simulink model "rlOvertakeTwoCars"  (R2022b)
settings: Solver=ode45  StartTime=0.0  StopTime=inf  FixedStep=0.001  RelTol=5e-3
PreLoadFcn:
  | setUpModel
PostLoadFcn:
  | setUpMain
model workspace (MAT data in the model file):
  firstWarning = 0
  originalScenarioChecksum = 'F73A6DA3C723D3CA73A6F931B7A52A9C'
values from neighbouring files (symbols this model uses):
  accel_vec = (-4:0.5:4)'    [setUpModel.m]
  amax = 3    [setUpMain.m]
  amin = -3    [setUpMain.m]
  dyNorm = [dyNorm 1.1]    [setUpSlipstream.m]
  e1_initial = 0    [setUpMain.m]
  e2_initial = 0    [setUpMain.m]
  L = data.ActorSpecifications.Length    [setUpModel.m]
  psi_o1 = 0.0058 * (pi/180)    (= 0.000101229096616)    [setUpModel.m]
  psi_o2 = 0.3528 *(pi/180)    (= 0.00615752160104)    [setUpModel.m]
  ry = [ry 0]    [setUpSlipstream.m]
  ssSwitch = 1    [setUpSlipstream.m]
  tolpsi = 10 * pi/180    (= 0.174532925199)    [setUpSlipstream.m]
  toly = 1.2*W /2    [setUpSlipstream.m]
  Ts = 0.1    [setUpMPC.m]
  TsRL = Ts    [setUpRLEnv.m]
  umax = 0.3    [setUpMain.m]
  umin = -0.3    [setUpMain.m]
  v_o1 = highSpeed1    (= 35)    [setUpModel.m]
  v_o2 = highSpeed2    (= 36)    [setUpModel.m]
  vel1 = highSpeed1 * ones(length(xlt),length(ylt))    [setUpModel.m]
  vel2 = highSpeed2 * ones(length(xlt),length(ylt))    [setUpModel.m]
  vel_vec = 0:2:20    [setUpModel.m]
  W = data.ActorSpecifications(1,1).Width    [setUpSlipstream.m]
  X_o1 = xRef1(1)    [setUpModel.m]
  X_o2 = xRef2(1)    [setUpModel.m]
  xFollow = [0 x1 xFollow 60]    [setUpSlipstream.m]
  xLead = [0 -x0 xLead]    [setUpSlipstream.m]
  xlt = -250:10:200    [setUpModel.m]
  Y_o1 = yRef1(1)    [setUpModel.m]
  Y_o2 = yRef2(1)    [setUpModel.m]
  yFollow = [c y1 yFollow 1]    [setUpSlipstream.m]
  yLead = [c y0 yLead]    [setUpSlipstream.m]
  ylt = -150:10:100    [setUpModel.m]
undefined symbols (not defined in the file or in its folder): curvature1, curvature2, deg, DiscIntNeverNeededParam, gradbp1, gradbp2, psi, rad, s, v_o, x_colpen, x_o, y_colpen, Z_colpen
libraries: simulink x26, autolibsharedcommon x22, autolibutils x10, autolibshared x10, vehdynlibtirecommon x8, drivingscenarioandsensors x4, autolibpowerinfoutils x4, sharedtransform x4, aerolibconvert2 x2, simulink_extras x2, vehdynlibtire x2, mpcadaslib x1
(part 1 of 8)
settings Model: PacingRate=0.700000  Creator=valakshe  LastModifiedBy=16koc1
settings SolverCC: AlgebraicLoopSolver=TrustRegion
settings DebuggingCC: UnconnectedInputMsg=warning  UnconnectedOutputMsg=warning  UnconnectedLineMsg=warning  SFMachineParentedDataDiag=warning
settings ModelReferenceCC: EnableRefExpFcnMdlSchedulingChecks=on
settings RTWCC: DLArmComputeVersion=19.05

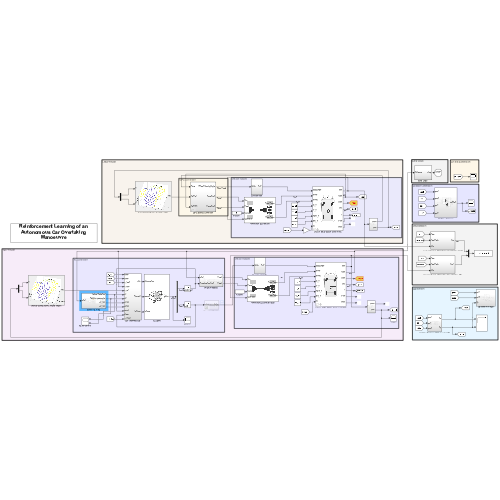
[thumbnail: Simulink's stored preview of the top-level diagram]
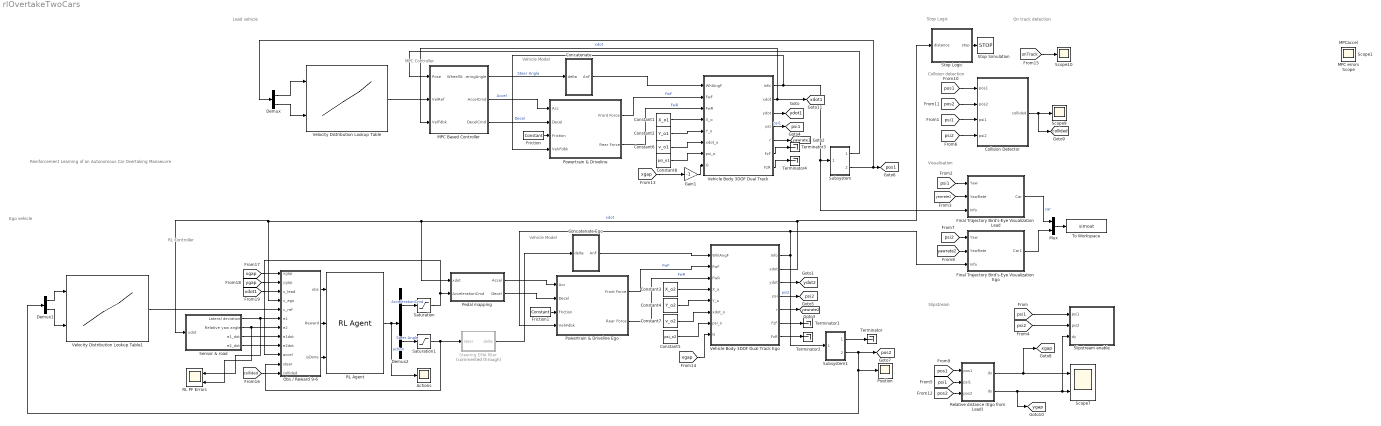
== system rlOvertakeTwoCars ==
  note: On track detection
  note: RL Controller
  note: Collision detection
  note: Slipstream
  note: Visualisation
  note: Ego vehicle
  note: Lead vehicle
  note: Stop Logic
  note: Vehicle Model
  note: Reinforcement Learning of an Autonomous Car Overtaking Manoeuvre
  note: MPC Controller
  note: Vehicle Model
  Actions : Scope
  Collision Detector : Subsystem
  Concatenate : Subsystem
  Concatenate Ego : Subsystem
  Constant1 : Constant  Value=X_o1
  Constant2 : Constant  Value=Y_o1
  Constant3 : Constant  Value=X_o2
  Constant4 : Constant  Value=Y_o2
  Constant5 : Constant  Value=psi_o2
  Constant6 : Constant  Value=v_o1
  Constant7 : Constant  Value=v_o2
  Constant8 : Constant  Value=psi_o1
  Demux : Demux  Outputs=2
  Demux1 : Demux  Outputs=2
  Demux2 : Demux  Outputs=2
  Final Trajectory Bird's-Eye Visualization Ego : Subsystem
  Final Trajectory Bird's-Eye Visualization Lead : Subsystem
  Friction : vehdynlibtirecommon/Constant  const=1.5  numWheels=4
  Friction1 : vehdynlibtirecommon/Constant  const=1.5  numWheels=4
  Gain1 : Gain  Gain=-1
  MPC Based Controller : Subsystem  AncestorBlock=rewardLibrary/MPC Based Controller  VariantControl=Stanley
      settings: LibrarySourceBlock=rewardLibrary/MPC Based Controller
  Mux : Mux  Inputs=2
  Obs / Reward 9-6 : Subsystem  AncestorBlock=rewardLibrary/Obs // Reward 6-2
      settings: LibrarySourceBlock=rewardLibrary/Obs // Reward 6-2
  Pedal mapping : Subsystem
  Position : Scope
  Powertrain & Driveline : Subsystem
      mask Display: image('vdbslibpt.png');
  Powertrain & Driveline Ego : Subsystem
      mask Display: image('vdbslibpt.png');
  RL Agent : rllib/RL Agent  Agent=agent  ExternalActionAsInput=off  ProvideLastAction=off  ProvideCumRwd=off  TreatAsDirectFeedthrough=on  UseStrictObservationDataTypes=off
  RL PF Errors : Scope  NumInputPorts=2
  Relative distance (Ego from Lead) : Subsystem
  Saturation : Saturate  UpperLimit=amax  LowerLimit=amin
  Saturation1 : Saturate  UpperLimit=umax  LowerLimit=umin
  Scope{,1,9..10} (4 alike) : Scope
  Scope7 : Scope  NumInputPorts=2
  Sensor & road : Subsystem
  Slipstream enable : Subsystem
  Steering EMA filter : Subsystem  Commented=through
  Stop Logic : Subsystem
  Stop Simulation : Stop
  Subsystem : Subsystem
  Subsystem1 : Subsystem
  Terminator{,1..4} (5 alike) : Terminator
  To Workspace : ToWorkspace  VariableName=simout  SaveFormat=Timeseries  SampleTime=-1
  Vehicle Body 3DOF Dual Track : Subsystem  AncestorBlock=autolibshared/Vehicle Body 3DOF Single Track  mask(Vehicle Body 3DOF Lateral){trackMode=Dual, inputMode=External forces, frontSteerMode=on, rearSteerMode=off, windMode=off, muMode=off, extFMode=off, extMMode=off, htchFMode=off, htchMMode=off, extXo=on, extpsio=on, extxdoto=on, extro=off, extYo=on, extTamb=off, extydoto=off, aMode=2, NF=2, NR=2, m=2000, a=1.4*4.7/3, b=1.6*4.7/3, h=0.35, dh=1, hh=0.2, X_o=0, xdot_o=v_o, CalphaMode=off, sigmaMode=on, d=0, hl=0, w=[1.4,1.4], Cy_f=12e3, Cy_r=11e3, sigma_f=.1, sigma_r=.1, alpha_f_brk=[-.1 .1], Cy_f_data=[-9e3 9e3], alpha_r_brk=[-.1 .1], Cy_r_data=[-9e3 9e3], Y_o=0, ydot_o=0, Izz=4000, psi_o=0, r_o=0, Af=2, Cd=.3, Cl=.1, Cpm=.1, beta_w=[0:0.01:0.3], Cs=[0:0.03:0.9], Cym=[0:0.01:0.3], Pabs=101325, Tair=273, g=9.81, mu=1, xdot_tol=.01, Fznom=5000, Fxtire_sat=7e4, Fytire_sat=7e4, longOff=0, latOff=0, vertOff=0, wrapAng=off}
      mask prompts: trackMode "autoblks_shared:autoblkVehBody3DofLat:blkPrm_trackMode"; inputMode "autoblks_shared:autoblkVehBody3DofLat:blkPrm_inputMode"; frontSteerMode "autoblks_shared:autoblkVehBody3DofLat:blkPrm_frontSteerMode"; rearSteerMode "autoblks_shared:autoblkVehBody3DofLat:blkPrm_rearSteerMode"; windMode "autoblks_shared:autoblkVehBody3DofLat:blkPrm_windMode"; muMode "autoblks_shared:autoblkVehBody3DofLat:blkPrm_muMode"; extFMode "autoblks_shared:autoblkVehBody3DofLat:blkPrm_extFMode"; extMMode "autoblks_shared:autoblkVehBody3DofLat:blkPrm_extMMode"; htchFMode "autoblks_shared:autoblkVehBody3DofLat:blkPrm_htchFMode"; htchMMode "autoblks_shared:autoblkVehBody3DofLat:blkPrm_htchMMode"; extXo "autoblks_shared:autoblkVehBody3DofLat:blkPrm_extXo"; extpsio "autoblks_shared:autoblkVehBody3DofLat:blkPrm_extpsio"; extxdoto "autoblks_shared:autoblkVehBody3DofLat:blkPrm_extxdoto"; extro "autoblks_shared:autoblkVehBody3DofLat:blkPrm_extro"; extYo "autoblks_shared:autoblkVehBody3DofLat:blkPrm_extYo"; extTamb "autoblks_shared:autoblkVehBody3DofLat:blkPrm_extTamb"; extydoto "autoblks_shared:autoblkVehBody3DofLat:blkPrm_extydoto"; NF "autoblks_shared:autoblkVehBody3DofLat:blkPrm_NF"; NR "autoblks_shared:autoblkVehBody3DofLat:blkPrm_NR"; m "autoblks_shared:autoblkVehBody3DofLat:blkPrm_m"; a "autoblks_shared:autoblkVehBody3DofLat:blkPrm_a"; b "autoblks_shared:autoblkVehBody3DofLat:blkPrm_b"; h "autoblks_shared:autoblkVehBody3DofLat:blkPrm_h"; dh "autoblks_shared:autoblkVehBody3DofLat:blkPrm_dh"; hh "autoblks_shared:autoblkVehBody3DofLat:blkPrm_hh"; X_o "autoblks_shared:autoblkVehBody3DofLat:blkPrm_X_o"; xdot_o "autoblks_shared:autoblkVehBody3DofLat:blkPrm_xdot_o"; CalphaMode "autoblks_shared:autoblkVehBody3DofLat:blkPrm_CalphaMode"; sigmaMode "autoblks_shared:autoblkVehBody3DofLat:blkPrm_sigmaMode"; d "autoblks_shared:autoblkVehBody3DofLat:blkPrm_d"; hl "autoblks_shared:autoblkVehBody3DofLat:blkPrm_hl"; w "autoblks_shared:autoblkVehBody3DofLat:blkPrm_w"; Cy_f "autoblks_shared:autoblkVehBody3DofLat:blkPrm_Cy_f"; Cy_r "autoblks_shared:autoblkVehBody3DofLat:blkPrm_Cy_r"; sigma_f "autoblks_shared:autoblkVehBody3DofLat:blkPrm_sigma_f"; sigma_r "autoblks_shared:autoblkVehBody3DofLat:blkPrm_sigma_r"; alpha_f_brk "autoblks_shared:autoblkVehBody3DofLat:blkPrm_alpha_f_brk"; Cy_f_data "autoblks_shared:autoblkVehBody3DofLat:blkPrm_Cy_f_data"; alpha_r_brk "autoblks_shared:autoblkVehBody3DofLat:blkPrm_alpha_r_brk"; Cy_r_data "autoblks_shared:autoblkVehBody3DofLat:blkPrm_Cy_r_data"; Y_o "autoblks_shared:autoblkVehBody3DofLat:blkPrm_Y_o"; ydot_o "autoblks_shared:autoblkVehBody3DofLat:blkPrm_ydot_o"; Izz "autoblks_shared:autoblkVehBody3DofLat:blkPrm_Izz"; psi_o "autoblks_shared:autoblkVehBody3DofLat:blkPrm_psi_o"; r_o "autoblks_shared:autoblkVehBody3DofLat:blkPrm_r_o"; Af "autoblks_shared:autoblkVehBody3DofLat:blkPrm_Af"; Cd "autoblks_shared:autoblkVehBody3DofLat:blkPrm_Cd"; Cl "autoblks_shared:autoblkVehBody3DofLat:blkPrm_Cl"; Cpm "autoblks_shared:autoblkVehBody3DofLat:blkPrm_Cpm"; beta_w "autoblks_shared:autoblkVehBody3DofLat:blkPrm_beta_w"; Cs "autoblks_shared:autoblkVehBody3DofLat:blkPrm_Cs"; Cym "autoblks_shared:autoblkVehBody3DofLat:blkPrm_Cym"; Pabs "autoblks_shared:autoblkVehBody3DofLat:blkPrm_Pabs"; Tair "autoblks_shared:autoblkVehBody3DofLat:blkPrm_Tair"; g "autoblks_shared:autoblkVehBody3DofLat:blkPrm_g"; mu "autoblks_shared:autoblkVehBody3DofLat:blkPrm_mu"; xdot_tol "autoblks_shared:autoblkVehBody3DofLat:blkPrm_xdot_tol"; Fznom "autoblks_shared:autoblkVehBody3DofLat:blkPrm_Fznom"; Fxtire_sat "autoblks_shared:autoblkVehBody3DofLat:blkPrm_Fxtire_sat"; Fytire_sat "autoblks_shared:autoblkVehBody3DofLat:blkPrm_Fytire_sat"; longOff "autoblks_shared:autoblkVehBody3DofLat:blkPrm_longOff"; latOff "autoblks_shared:autoblkVehBody3DofLat:blkPrm_latOff"; vertOff "autoblks_shared:autoblkVehBody3DofLat:blkPrm_vertOff"; wrapAng "autoblks_shared:autoblkVehBody3DofLat:blkPrm_wrapAng"
      mask help: autoblks_shared:autoblkVehBody3DofLat:blkDesc
      mask init:
      | [~]=autosharedicon('vehdynliblat3dof',gcb,0);
      settings: LibrarySourceBlock=autolibshared/Vehicle Body 3DOF Single Track
      mask Help: eval('autosharedhelp(''vb3doflat'')');
      mask TypeOptions trackMode: autoblks_shared:autoblkVehBody3DofLat:blkCmb_trackMode_c1 | autoblks_shared:autoblkVehBody3DofLat:blkCmb_trackMode_c2
      mask Callback trackMode: [~]=autosharedicon('vehdynliblat3dof',gcb,5);
      mask TypeOptions inputMode: autoblks_shared:autoblkVehBody3DofLat:blkCmb_inputMode_c1 | autoblks_shared:autoblkVehBody3DofLat:blkCmb_inputMode_c2 | autoblks_shared:autoblkVehBody3DofLat:blkCmb_inputMode_c3
      mask Callback inputMode: [~]=autosharedicon('vehdynliblat3dof',gcb,1);
      mask Callback muMode: [~]=autosharedicon('vehdynliblat3dof',gcb,2);
      mask Callback extXo: [~]=autosharedicon('vehdynliblat3dof',gcb,7);
      mask Callback extpsio: [~]=autosharedicon('vehdynliblat3dof',gcb,7);
      mask Callback extxdoto: [~]=autosharedicon('vehdynliblat3dof',gcb,7);
      mask Callback extro: [~]=autosharedicon('vehdynliblat3dof',gcb,7);
      mask Callback extYo: [~]=autosharedicon('vehdynliblat3dof',gcb,7);
      mask Callback extTamb: [~]=autosharedicon('vehdynliblat3dof',gcb,6);
      mask Callback extydoto: [~]=autosharedicon('vehdynliblat3dof',gcb,7);
      mask Callback CalphaMode: [~]=autosharedicon('vehdynliblat3dof',gcb,3);
      mask Callback sigmaMode: [~]=autosharedicon('vehdynliblat3dof',gcb,4);
      mask DialogControl blockConfig Prompt: autoblks_shared:autoblkVehBody3DofLat:blkDlg_blockConfig
      mask DialogControl trackMode Prompt: Vehicle track:
      mask DialogControl inputMode Prompt: Axle forces:
      mask DialogControl extModePanel Prompt: autoblks_shared:autoblkVehBody3DofLat:blkDlg_extModePanel
      mask DialogControl frontSteerMode Prompt: Front wheel steering
      mask DialogControl rearSteerMode Prompt: Rear wheel steering
      mask DialogControl windMode Prompt: External wind
      mask DialogControl muMode Prompt: External friction
      mask DialogControl extFMode Prompt: External forces
      mask DialogControl extMMode Prompt: External moments
      mask DialogControl htchFMode Prompt: Hitch forces
      mask DialogControl htchMMode Prompt: Hitch moments
      mask DialogControl extXo Prompt: Initial longitudinal position
      mask DialogControl extpsio Prompt: Initial yaw angle
      mask DialogControl extxdoto Prompt: Initial longitudinal velocity
      mask DialogControl extro Prompt: Initial yaw rate
      mask DialogControl extYo Prompt: Initial lateral position
      mask DialogControl extTamb Prompt: Air temperature
      mask DialogControl extydoto Prompt: Initial lateral velocity
      mask DialogControl ParameterGroupVar Prompt: autoblks_shared:autoblkVehBody3DofLat:blkDlg_ParameterGroupVar
      mask DialogControl LongPanel Prompt: autoblks_shared:autoblkVehBody3DofLat:blkDlg_LongPanel
      mask DialogControl NF Prompt: Number of wheels on front axle, NF [-]:
      mask DialogControl NR Prompt: Number of wheels on rear axle, NR [-]:
      mask DialogControl m Prompt: Vehicle mass, m [kg]:
      mask DialogControl a Prompt: Longitudinal distance from center of mass to front axle, a [m]:
      mask DialogControl b Prompt: Longitudinal distance from center of mass to rear axle, b [m]:
      mask DialogControl h Prompt: Vertical distance from center of mass to axle plane, h [m]:
      mask DialogControl dh Prompt: Longitudinal distance from center of mass to hitch, dh [m]:
      mask DialogControl hh Prompt: Vertical distance from hitch to axle plane, hh [m]:
      mask DialogControl X_o Prompt: Initial inertial frame longitudinal position, X_o [m]:
      mask DialogControl xdot_o Prompt: Initial longitudinal velocity, xdot_o [m/s]:
      mask DialogControl LatPanel Prompt: autoblks_shared:autoblkVehBody3DofLat:blkDlg_LatPanel
      mask DialogControl CalphaMode Prompt: Mapped corner stiffness:
      mask DialogControl sigmaMode Prompt: Include relaxation length dynamics:
      mask DialogControl d Prompt: Lateral distance from geometric centerline to center of mass, d [m]:
      mask DialogControl hl Prompt: Lateral distance from geometric centerline to hitch, hl [m]:
      mask DialogControl w Prompt: Track width, w [m]:
      mask DialogControl Cy_f Prompt: Front tire corner stiffness, Cy_f [N/rad]:
      mask DialogControl Cy_r Prompt: Rear tire axle corner stiffness, Cy_r [N/rad]:
      mask DialogControl sigma_f Prompt: Front tire(s) relaxation length, sigma_f [m]:
      mask DialogControl sigma_r Prompt: Rear tire(s) relaxation length, sigma_r [m]:
      mask DialogControl alpha_f_brk Prompt: Front axle slip angle breakpoints, alpha_f_brk [rad]:
      mask DialogControl Cy_f_data Prompt: Front axle corner data, Cy_f_data [N/rad]:
      mask DialogControl alpha_r_brk Prompt: Rear axle slip angle breakpoints, alpha_r_brk [rad]:
      mask DialogControl Cy_r_data Prompt: Rear axle corner data, Cy_r_data [N/rad]:
      mask DialogControl Y_o Prompt: Initial inertial frame lateral displacement, Y_o [m]:
      mask DialogControl ydot_o Prompt: Initial lateral velocity, ydot_o [m/s]:
      mask DialogControl YawPanel Prompt: autoblks_shared:autoblkVehBody3DofLat:blkDlg_YawPanel
      mask DialogControl Izz Prompt: Yaw polar inertia, Izz [kg*m^2]:
      mask DialogControl psi_o Prompt: Initial yaw angle, psi_o [rad]:
      mask DialogControl r_o Prompt: Initial yaw rate, r_o [rad/s]:
      mask DialogControl AeroParams Prompt: autoblks_shared:autoblkVehBody3DofLat:blkDlg_AeroParams
      mask DialogControl Af Prompt: Longitudinal drag area, Af [m^2]:
      mask DialogControl Cd Prompt: Longitudinal drag coefficient, Cd [-]:
      mask DialogControl Cl Prompt: Longitudinal lift coefficient, Cl [-]:
      mask DialogControl Cpm Prompt: Longitudinal drag pitch moment, Cpm [-]:
      mask DialogControl beta_w Prompt: Relative wind angle vector, beta_w [rad]:
      mask DialogControl Cs Prompt: Side force coefficient vector, Cs [-]:
      mask DialogControl Cym Prompt: Yaw moment coefficient vector, Cym [-]:
      mask DialogControl EnviroPanel Prompt: autoblks_shared:autoblkVehBody3DofLat:blkDlg_EnviroPanel
      mask DialogControl Pabs Prompt: Absolute pressure, Pabs [Pa]:
      mask DialogControl Tair Prompt: Air temperature, Tair [K]:
      mask DialogControl g Prompt: Gravitational acceleration, g [m/s^2]:
      mask DialogControl mu Prompt: Nominal friction scaling factor, mu [-]:
      mask DialogControl SimPanel Prompt: autoblks_shared:autoblkVehBody3DofLat:blkDlg_SimPanel
      mask DialogControl xdot_tol Prompt: Longitudinal velocity tolerance, xdot_tol [m/s]:
      mask DialogControl Fznom Prompt: Nominal normal force, Fznom [N]:
      mask DialogControl Fxtire_sat Prompt: Longitudinal force limit, Fxtire_sat [N]:
      mask DialogControl Fytire_sat Prompt: Lateral force limit, Fytire_sat [N]:
      mask DialogControl longOff Prompt: Geometric longitudinal offset from axle plane, longOff [m]:
      mask DialogControl latOff Prompt: Geometric lateral offset from center plane, latOff [m]:
      mask DialogControl vertOff Prompt: Geometric vertical offset from axle plane, vertOff [m]:
      mask DialogControl wrapAng Prompt: Wrap Euler angles, wrapAng
      mask Display:
      | try
      |     IconInfo = autosharedicon('vehdynliblat3dof',gcb,8);
      | 
      |     image(IconInfo.image, IconInfo.position);
      | 
      |     for i = 1:numel(IconInfo.lconn)
      |         port_label('lconn', i, IconInfo.lconn{i})
      |     end
      | 
      |     for j = 1:numel(IconInfo.rconn)
      |         port_label('rconn', j, IconInfo.rconn{j})
      |     end
      | 
      |     for k = 1:numel(IconInfo.input)
      |         port_label('input', k, IconInfo.input{k})
      |     end
      | 
      |     for m = 1:numel(IconInfo.output)
      |         port_label('output', m, IconInfo.output{m})
      |     end
      | catch
      |     fprintf('Vehicle Body \n 3DOF Lateral')
      | end
  Vehicle Body 3DOF Dual Track Ego : Subsystem  AncestorBlock=autolibshared/Vehicle Body 3DOF Single Track  mask(Vehicle Body 3DOF Lateral){trackMode=Dual, inputMode=External forces, frontSteerMode=on, rearSteerMode=off, windMode=off, muMode=off, extFMode=off, extMMode=off, htchFMode=off, htchMMode=off, extXo=on, extpsio=on, extxdoto=on, extro=off, extYo=on, extTamb=off, extydoto=off, aMode=2, NF=2, NR=2, m=2000, a=1.4*4.7/3, b=1.6*4.7/3, h=0.35, dh=1, hh=0.2, X_o=0, xdot_o=v_o, CalphaMode=off, sigmaMode=on, d=0, hl=0, w=[1.4,1.4], Cy_f=12e3, Cy_r=11e3, sigma_f=.1, sigma_r=.1, alpha_f_brk=[-.1 .1], Cy_f_data=[-9e3 9e3], alpha_r_brk=[-.1 .1], Cy_r_data=[-9e3 9e3], Y_o=0, ydot_o=0, Izz=4000, psi_o=0, r_o=0, Af=2, Cd=.3, Cl=.1, Cpm=.1, beta_w=[0:0.01:0.3], Cs=[0:0.03:0.9], Cym=[0:0.01:0.3], Pabs=101325, Tair=273, g=9.81, mu=1, xdot_tol=.01, Fznom=5000, Fxtire_sat=7e4, Fytire_sat=7e4, longOff=0, latOff=0, vertOff=0, wrapAng=off}
      mask prompts: trackMode "autoblks_shared:autoblkVehBody3DofLat:blkPrm_trackMode"; inputMode "autoblks_shared:autoblkVehBody3DofLat:blkPrm_inputMode"; frontSteerMode "autoblks_shared:autoblkVehBody3DofLat:blkPrm_frontSteerMode"; rearSteerMode "autoblks_shared:autoblkVehBody3DofLat:blkPrm_rearSteerMode"; windMode "autoblks_shared:autoblkVehBody3DofLat:blkPrm_windMode"; muMode "autoblks_shared:autoblkVehBody3DofLat:blkPrm_muMode"; extFMode "autoblks_shared:autoblkVehBody3DofLat:blkPrm_extFMode"; extMMode "autoblks_shared:autoblkVehBody3DofLat:blkPrm_extMMode"; htchFMode "autoblks_shared:autoblkVehBody3DofLat:blkPrm_htchFMode"; htchMMode "autoblks_shared:autoblkVehBody3DofLat:blkPrm_htchMMode"; extXo "autoblks_shared:autoblkVehBody3DofLat:blkPrm_extXo"; extpsio "autoblks_shared:autoblkVehBody3DofLat:blkPrm_extpsio"; extxdoto "autoblks_shared:autoblkVehBody3DofLat:blkPrm_extxdoto"; extro "autoblks_shared:autoblkVehBody3DofLat:blkPrm_extro"; extYo "autoblks_shared:autoblkVehBody3DofLat:blkPrm_extYo"; extTamb "autoblks_shared:autoblkVehBody3DofLat:blkPrm_extTamb"; extydoto "autoblks_shared:autoblkVehBody3DofLat:blkPrm_extydoto"; NF "autoblks_shared:autoblkVehBody3DofLat:blkPrm_NF"; NR "autoblks_shared:autoblkVehBody3DofLat:blkPrm_NR"; m "autoblks_shared:autoblkVehBody3DofLat:blkPrm_m"; a "autoblks_shared:autoblkVehBody3DofLat:blkPrm_a"; b "autoblks_shared:autoblkVehBody3DofLat:blkPrm_b"; h "autoblks_shared:autoblkVehBody3DofLat:blkPrm_h"; dh "autoblks_shared:autoblkVehBody3DofLat:blkPrm_dh"; hh "autoblks_shared:autoblkVehBody3DofLat:blkPrm_hh"; X_o "autoblks_shared:autoblkVehBody3DofLat:blkPrm_X_o"; xdot_o "autoblks_shared:autoblkVehBody3DofLat:blkPrm_xdot_o"; CalphaMode "autoblks_shared:autoblkVehBody3DofLat:blkPrm_CalphaMode"; sigmaMode "autoblks_shared:autoblkVehBody3DofLat:blkPrm_sigmaMode"; d "autoblks_shared:autoblkVehBody3DofLat:blkPrm_d"; hl "autoblks_shared:autoblkVehBody3DofLat:blkPrm_hl"; w "autoblks_shared:autoblkVehBody3DofLat:blkPrm_w"; Cy_f "autoblks_shared:autoblkVehBody3DofLat:blkPrm_Cy_f"; Cy_r "autoblks_shared:autoblkVehBody3DofLat:blkPrm_Cy_r"; sigma_f "autoblks_shared:autoblkVehBody3DofLat:blkPrm_sigma_f"; sigma_r "autoblks_shared:autoblkVehBody3DofLat:blkPrm_sigma_r"; alpha_f_brk "autoblks_shared:autoblkVehBody3DofLat:blkPrm_alpha_f_brk"; Cy_f_data "autoblks_shared:autoblkVehBody3DofLat:blkPrm_Cy_f_data"; alpha_r_brk "autoblks_shared:autoblkVehBody3DofLat:blkPrm_alpha_r_brk"; Cy_r_data "autoblks_shared:autoblkVehBody3DofLat:blkPrm_Cy_r_data"; Y_o "autoblks_shared:autoblkVehBody3DofLat:blkPrm_Y_o"; ydot_o "autoblks_shared:autoblkVehBody3DofLat:blkPrm_ydot_o"; Izz "autoblks_shared:autoblkVehBody3DofLat:blkPrm_Izz"; psi_o "autoblks_shared:autoblkVehBody3DofLat:blkPrm_psi_o"; r_o "autoblks_shared:autoblkVehBody3DofLat:blkPrm_r_o"; Af "autoblks_shared:autoblkVehBody3DofLat:blkPrm_Af"; Cd "autoblks_shared:autoblkVehBody3DofLat:blkPrm_Cd"; Cl "autoblks_shared:autoblkVehBody3DofLat:blkPrm_Cl"; Cpm "autoblks_shared:autoblkVehBody3DofLat:blkPrm_Cpm"; beta_w "autoblks_shared:autoblkVehBody3DofLat:blkPrm_beta_w"; Cs "autoblks_shared:autoblkVehBody3DofLat:blkPrm_Cs"; Cym "autoblks_shared:autoblkVehBody3DofLat:blkPrm_Cym"; Pabs "autoblks_shared:autoblkVehBody3DofLat:blkPrm_Pabs"; Tair "autoblks_shared:autoblkVehBody3DofLat:blkPrm_Tair"; g "autoblks_shared:autoblkVehBody3DofLat:blkPrm_g"; mu "autoblks_shared:autoblkVehBody3DofLat:blkPrm_mu"; xdot_tol "autoblks_shared:autoblkVehBody3DofLat:blkPrm_xdot_tol"; Fznom "autoblks_shared:autoblkVehBody3DofLat:blkPrm_Fznom"; Fxtire_sat "autoblks_shared:autoblkVehBody3DofLat:blkPrm_Fxtire_sat"; Fytire_sat "autoblks_shared:autoblkVehBody3DofLat:blkPrm_Fytire_sat"; longOff "autoblks_shared:autoblkVehBody3DofLat:blkPrm_longOff"; latOff "autoblks_shared:autoblkVehBody3DofLat:blkPrm_latOff"; vertOff "autoblks_shared:autoblkVehBody3DofLat:blkPrm_vertOff"; wrapAng "autoblks_shared:autoblkVehBody3DofLat:blkPrm_wrapAng"
      mask help: autoblks_shared:autoblkVehBody3DofLat:blkDesc
      mask init:
      | [~]=autosharedicon('vehdynliblat3dof',gcb,0);
      settings: LibrarySourceBlock=autolibshared/Vehicle Body 3DOF Single Track
      mask Help: eval('autosharedhelp(''vb3doflat'')');
      mask TypeOptions trackMode: autoblks_shared:autoblkVehBody3DofLat:blkCmb_trackMode_c1 | autoblks_shared:autoblkVehBody3DofLat:blkCmb_trackMode_c2
      mask Callback trackMode: [~]=autosharedicon('vehdynliblat3dof',gcb,5);
      mask TypeOptions inputMode: autoblks_shared:autoblkVehBody3DofLat:blkCmb_inputMode_c1 | autoblks_shared:autoblkVehBody3DofLat:blkCmb_inputMode_c2 | autoblks_shared:autoblkVehBody3DofLat:blkCmb_inputMode_c3
      mask Callback inputMode: [~]=autosharedicon('vehdynliblat3dof',gcb,1);
      mask Callback muMode: [~]=autosharedicon('vehdynliblat3dof',gcb,2);
      mask Callback extXo: [~]=autosharedicon('vehdynliblat3dof',gcb,7);
      mask Callback extpsio: [~]=autosharedicon('vehdynliblat3dof',gcb,7);
      mask Callback extxdoto: [~]=autosharedicon('vehdynliblat3dof',gcb,7);
      mask Callback extro: [~]=autosharedicon('vehdynliblat3dof',gcb,7);
      mask Callback extYo: [~]=autosharedicon('vehdynliblat3dof',gcb,7);
      mask Callback extTamb: [~]=autosharedicon('vehdynliblat3dof',gcb,6);
      mask Callback extydoto: [~]=autosharedicon('vehdynliblat3dof',gcb,7);
      mask Callback CalphaMode: [~]=autosharedicon('vehdynliblat3dof',gcb,3);
      mask Callback sigmaMode: [~]=autosharedicon('vehdynliblat3dof',gcb,4);
      mask DialogControl blockConfig Prompt: autoblks_shared:autoblkVehBody3DofLat:blkDlg_blockConfig
      mask DialogControl trackMode Prompt: Vehicle track:
      mask DialogControl inputMode Prompt: Axle forces:
      mask DialogControl extModePanel Prompt: autoblks_shared:autoblkVehBody3DofLat:blkDlg_extModePanel
      mask DialogControl frontSteerMode Prompt: Front wheel steering
      mask DialogControl rearSteerMode Prompt: Rear wheel steering
      mask DialogControl windMode Prompt: External wind
      mask DialogControl muMode Prompt: External friction
      mask DialogControl extFMode Prompt: External forces
      mask DialogControl extMMode Prompt: External moments
      mask DialogControl htchFMode Prompt: Hitch forces
      mask DialogControl htchMMode Prompt: Hitch moments
      mask DialogControl extXo Prompt: Initial longitudinal position
      mask DialogControl extpsio Prompt: Initial yaw angle
      mask DialogControl extxdoto Prompt: Initial longitudinal velocity
      mask DialogControl extro Prompt: Initial yaw rate
      mask DialogControl extYo Prompt: Initial lateral position
      mask DialogControl extTamb Prompt: Air temperature
      mask DialogControl extydoto Prompt: Initial lateral velocity
      mask DialogControl ParameterGroupVar Prompt: autoblks_shared:autoblkVehBody3DofLat:blkDlg_ParameterGroupVar
      mask DialogControl LongPanel Prompt: autoblks_shared:autoblkVehBody3DofLat:blkDlg_LongPanel
      mask DialogControl NF Prompt: Number of wheels on front axle, NF [-]:
      mask DialogControl NR Prompt: Number of wheels on rear axle, NR [-]:
      mask DialogControl m Prompt: Vehicle mass, m [kg]:
      mask DialogControl a Prompt: Longitudinal distance from center of mass to front axle, a [m]:
      mask DialogControl b Prompt: Longitudinal distance from center of mass to rear axle, b [m]:
      mask DialogControl h Prompt: Vertical distance from center of mass to axle plane, h [m]:
      mask DialogControl dh Prompt: Longitudinal distance from center of mass to hitch, dh [m]:
      mask DialogControl hh Prompt: Vertical distance from hitch to axle plane, hh [m]:
      mask DialogControl X_o Prompt: Initial inertial frame longitudinal position, X_o [m]:
      mask DialogControl xdot_o Prompt: Initial longitudinal velocity, xdot_o [m/s]:
      mask DialogControl LatPanel Prompt: autoblks_shared:autoblkVehBody3DofLat:blkDlg_LatPanel
      mask DialogControl CalphaMode Prompt: Mapped corner stiffness:
      mask DialogControl sigmaMode Prompt: Include relaxation length dynamics:
      mask DialogControl d Prompt: Lateral distance from geometric centerline to center of mass, d [m]:
      mask DialogControl hl Prompt: Lateral distance from geometric centerline to hitch, hl [m]:
      mask DialogControl w Prompt: Track width, w [m]:
      mask DialogControl Cy_f Prompt: Front tire corner stiffness, Cy_f [N/rad]:
      mask DialogControl Cy_r Prompt: Rear tire axle corner stiffness, Cy_r [N/rad]:
      mask DialogControl sigma_f Prompt: Front tire(s) relaxation length, sigma_f [m]:
      mask DialogControl sigma_r Prompt: Rear tire(s) relaxation length, sigma_r [m]:
      mask DialogControl alpha_f_brk Prompt: Front axle slip angle breakpoints, alpha_f_brk [rad]:
      mask DialogControl Cy_f_data Prompt: Front axle corner data, Cy_f_data [N/rad]:
      mask DialogControl alpha_r_brk Prompt: Rear axle slip angle breakpoints, alpha_r_brk [rad]:
      mask DialogControl Cy_r_data Prompt: Rear axle corner data, Cy_r_data [N/rad]:
      mask DialogControl Y_o Prompt: Initial inertial frame lateral displacement, Y_o [m]:
      mask DialogControl ydot_o Prompt: Initial lateral velocity, ydot_o [m/s]:
      mask DialogControl YawPanel Prompt: autoblks_shared:autoblkVehBody3DofLat:blkDlg_YawPanel
      mask DialogControl Izz Prompt: Yaw polar inertia, Izz [kg*m^2]:
      mask DialogControl psi_o Prompt: Initial yaw angle, psi_o [rad]:
      mask DialogControl r_o Prompt: Initial yaw rate, r_o [rad/s]:
      mask DialogControl AeroParams Prompt: autoblks_shared:autoblkVehBody3DofLat:blkDlg_AeroParams
      mask DialogControl Af Prompt: Longitudinal drag area, Af [m^2]:
      mask DialogControl Cd Prompt: Longitudinal drag coefficient, Cd [-]:
      mask DialogControl Cl Prompt: Longitudinal lift coefficient, Cl [-]:
      mask DialogControl Cpm Prompt: Longitudinal drag pitch moment, Cpm [-]:
      mask DialogControl beta_w Prompt: Relative wind angle vector, beta_w [rad]:
      mask DialogControl Cs Prompt: Side force coefficient vector, Cs [-]:
      mask DialogControl Cym Prompt: Yaw moment coefficient vector, Cym [-]:
      mask DialogControl EnviroPanel Prompt: autoblks_shared:autoblkVehBody3DofLat:blkDlg_EnviroPanel
      mask DialogControl Pabs Prompt: Absolute pressure, Pabs [Pa]:
      mask DialogControl Tair Prompt: Air temperature, Tair [K]:
      mask DialogControl g Prompt: Gravitational acceleration, g [m/s^2]:
      mask DialogControl mu Prompt: Nominal friction scaling factor, mu [-]:
      mask DialogControl SimPanel Prompt: autoblks_shared:autoblkVehBody3DofLat:blkDlg_SimPanel
      mask DialogControl xdot_tol Prompt: Longitudinal velocity tolerance, xdot_tol [m/s]:
      mask DialogControl Fznom Prompt: Nominal normal force, Fznom [N]:
      mask DialogControl Fxtire_sat Prompt: Longitudinal force limit, Fxtire_sat [N]:
      mask DialogControl Fytire_sat Prompt: Lateral force limit, Fytire_sat [N]:
      mask DialogControl longOff Prompt: Geometric longitudinal offset from axle plane, longOff [m]:
      mask DialogControl latOff Prompt: Geometric lateral offset from center plane, latOff [m]:
      mask DialogControl vertOff Prompt: Geometric vertical offset from axle plane, vertOff [m]:
      mask DialogControl wrapAng Prompt: Wrap Euler angles, wrapAng
      mask Display:
      | try
      |     IconInfo = autosharedicon('vehdynliblat3dof',gcb,8);
      | 
      |     image(IconInfo.image, IconInfo.position);
      | 
      |     for i = 1:numel(IconInfo.lconn)
      |         port_label('lconn', i, IconInfo.lconn{i})
      |     end
      | 
      |     for j = 1:numel(IconInfo.rconn)
      |         port_label('rconn', j, IconInfo.rconn{j})
      |     end
      | 
      |     for k = 1:numel(IconInfo.input)
      |         port_label('input', k, IconInfo.input{k})
      |     end
      | 
      |     for m = 1:numel(IconInfo.output)
      |         port_label('output', m, IconInfo.output{m})
      |     end
      | catch
      |     fprintf('Vehicle Body \n 3DOF Lateral')
      | end
  Velocity Distribution Lookup Table : Lookup_n-D  BreakpointsForDimension1=xlt  BreakpointsForDimension2=ylt  Table=vel1  ExtrapMethod=Clip  InternalRulePriority=Speed  RndMeth=Simplest
      settings: InputPortMap=u0,u1
      mask Display:
      | image("LookupTable.PNG")
      | port_label('input', 1, 'x')
      | port_label('input', 2, 'y')
      | port_label('output', 1, 'vel')
  Velocity Distribution Lookup Table1 : Lookup_n-D  BreakpointsForDimension1=xlt  BreakpointsForDimension2=ylt  Table=vel2  ExtrapMethod=Clip  InternalRulePriority=Speed  RndMeth=Simplest
      settings: InputPortMap=u0,u1
      mask Display:
      | image("LookupTable.PNG")
      | port_label('input', 1, 'x')
      | port_label('input', 2, 'y')
      | port_label('output', 1, 'vel')
  MPC errors : Scope
  MPCaccel : Scope
  tag scope: collided=global, pos1=global, pos2=global, psi1=global, psi2=global, xdot1=global, xgap=global, yawrate1=global, yawrate2=global, ydot1=global, ydot2=global, ygap=global
  wires:
  Vehicle Body 3DOF Dual Track/7(FzR) -> Terminator4/1
  Powertrain & Driveline/1(Front Force) -> Vehicle Body 3DOF Dual Track/2(FwF)  "FwF"
  Vehicle Body 3DOF Dual Track/1(Info) -> Final Trajectory Bird's-Eye Visualization Lead/3(Info), Subsystem/1(In1), Powertrain & Driveline/4(VehFdbk)
  Constant1/1 -> Vehicle Body 3DOF Dual Track/4(X_o)
  Vehicle Body 3DOF Dual Track/2(xdot) -> MPC Based Controller/3(VelFdbk), [xdot1]  "xdot"
  Vehicle Body 3DOF Dual Track/3(ydot) -> [ydot1]
  Concatenate/1(AnF) -> Vehicle Body 3DOF Dual Track/1(WhlAngF)
  Vehicle Body 3DOF Dual Track/6(FzF) -> Terminator3/1
  Constant8/1 -> Vehicle Body 3DOF Dual Track/7(psi_o)
  Powertrain & Driveline/2(Rear Force) -> Vehicle Body 3DOF Dual Track/3(FwR)  "FwR"
  Vehicle Body 3DOF Dual Track/5(r) -> [yawrate1]
  Constant2/1 -> Vehicle Body 3DOF Dual Track/5(Y_o)
  Friction/1 -> Powertrain & Driveline/3(Friction)
  Subsystem/1(pose) -> MPC Based Controller/1(Pose)
  MPC Based Controller/2(AccelCmd) -> Powertrain & Driveline/1(Acc)  "Accel"
  MPC Based Controller/3(DecelCmd) -> Powertrain & Driveline/2(Decel)  "Decel"
  MPC Based Controller/1(WheelSteeringAngle) -> Concatenate/1(delta)  "Steer Angle"
  Velocity Distribution Lookup Table/1 -> MPC Based Controller/2(VelRef)
  Stop Logic/1(stop) -> Stop Simulation/1
  Vehicle Body 3DOF Dual Track Ego/6(FzF) -> Terminator1/1
  Constant5/1 -> Vehicle Body 3DOF Dual Track Ego/7(psi_o)
  Vehicle Body 3DOF Dual Track Ego/1(Info) -> Subsystem1/1(In1), Final Trajectory Bird's-Eye Visualization Ego/3(Info), Powertrain & Driveline Ego/4(VehFdbk)
  Friction1/1 -> Powertrain & Driveline Ego/3(Friction)
  Constant4/1 -> Vehicle Body 3DOF Dual Track Ego/5(Y_o)
  Constant3/1 -> Vehicle Body 3DOF Dual Track Ego/4(X_o)
  Vehicle Body 3DOF Dual Track Ego/5(r) -> [yawrate2]
  Vehicle Body 3DOF Dual Track Ego/2(xdot) -> Sensor & road/1(xdot), Obs / Reward 9-6/4(v_ego), Pedal mapping/1(xdot), Stop Logic/1(distance)  "xdot"
  Concatenate Ego/1(AnF) -> Vehicle Body 3DOF Dual Track Ego/1(WhlAngF)
  Powertrain & Driveline Ego/1(Front Force) -> Vehicle Body 3DOF Dual Track Ego/2(FwF)  "FwF"
  Vehicle Body 3DOF Dual Track Ego/7(FzR) -> Terminator2/1
  Powertrain & Driveline Ego/2(Rear Force) -> Vehicle Body 3DOF Dual Track Ego/3(FwR)  "FwR"
  Vehicle Body 3DOF Dual Track Ego/3(ydot) -> [ydot2]
  Final Trajectory Bird's-Eye Visualization Lead/1(Car) -> Mux/1  "car"
  Final Trajectory Bird's-Eye Visualization Ego/1(Car1) -> Mux/2
  Mux/1 -> To Workspace/1
  Constant6/1 -> Vehicle Body 3DOF Dual Track/6(xdot_o)
  Constant7/1 -> Vehicle Body 3DOF Dual Track Ego/6(xdot_o)
  Relative distance (Ego from Lead)/2(dy) -> [ygap], Slipstream enable/3(dy), Scope7/2
  Gain1/1 -> Vehicle Body 3DOF Dual Track/8(G)
  Subsystem/2(pos) -> Demux/1, [pos1]
  Collision Detector/1(collided) -> [collided], Scope9/1
  Demux/1 -> Velocity Distribution Lookup Table/1
  Demux/2 -> Velocity Distribution Lookup Table/2
  Demux1/1 -> Velocity Distribution Lookup Table1/1
  Demux1/2 -> Velocity Distribution Lookup Table1/2
  Vehicle Body 3DOF Dual Track/4(psi) -> [psi1]  "psi1"
  [psi1] -> Slipstream enable/1(psi1)
  [psi1] -> Collision Detector/3(psi1)
  [psi1] -> Final Trajectory Bird's-Eye Visualization Lead/1(Yaw)
  [yawrate1] -> Final Trajectory Bird's-Eye Visualization Lead/2(YawRate)
  Vehicle Body 3DOF Dual Track Ego/4(psi) -> [psi2]  "psi2"
  [psi2] -> Slipstream enable/2(psi2)
  [psi1] -> Relative distance (Ego from Lead)/2(psi1)
  [psi2] -> Collision Detector/4(psi2)
  [psi2] -> Final Trajectory Bird's-Eye Visualization Ego/1(Yaw)
  [yawrate2] -> Final Trajectory Bird's-Eye Visualization Ego/2(YawRate)
  [pos1] -> Relative distance (Ego from Lead)/1(pos1)
  [pos1] -> Collision Detector/1(pos1)
  [pos2] -> Collision Detector/2(pos2)
  [pos2] -> Relative distance (Ego from Lead)/3(pos2)
  [xgap] -> Gain1/1
  [xgap] -> Vehicle Body 3DOF Dual Track Ego/8(G)
  Subsystem1/1(pose) -> Terminator/1
  Obs / Reward 9-6/1(obs) -> RL Agent/1
  Obs / Reward 9-6/3(isDone) -> RL Agent/3
  Obs / Reward 9-6/2(Reward) -> RL Agent/2
  RL Agent/1 -> Actions/1, Demux2/1  "action"
  Sensor & road/3(e1_dot) -> Obs / Reward 9-6/8(e1dot)
  Sensor & road/4(e2_dot) -> Obs / Reward 9-6/9(e2dot)
  Sensor & road/1(Lateral deviation) -> RL PF Errors/1, Obs / Reward 9-6/6(e1)
  Sensor & road/2(Relative yaw angle) -> Obs / Reward 9-6/7(e2), RL PF Errors/2
  Pedal mapping/1(Accel) -> Powertrain & Driveline Ego/1(Acc)
  Pedal mapping/2(Decel) -> Powertrain & Driveline Ego/2(Decel)
  [onTrack] -> Scope10/1
  Demux2/1 -> Saturation/1  "AccelerationCmd"
  Saturation/1 -> Obs / Reward 9-6/10(accel), Pedal mapping/2(AccelerationCmd)
  Demux2/2 -> Saturation1/1  "Steer Angle"
  Saturation1/1 -> Obs / Reward 9-6/11(steer), Steering EMA filter/1(steer)
  [collided] -> Obs / Reward 9-6/12(collided)
  [xgap] -> Obs / Reward 9-6/1(xgap)
  [ygap] -> Obs / Reward 9-6/2(ygap)
  [xdot1] -> Obs / Reward 9-6/3(v_lead)
  Velocity Distribution Lookup Table1/1 -> Obs / Reward 9-6/5(v_ref)
  Relative distance (Ego from Lead)/1(dx) -> [xgap], Scope7/1
  Steering EMA filter/1(delta) -> Concatenate Ego/1(delta)
  Subsystem1/2(pos) -> Demux1/1, Position/1, [pos2]

== system rlOvertakeTwoCars/Collision Detector ==
  pos1 : Inport
  pos2 : Inport  Port=2
  psi1 : Inport  Port=3
  psi2 : Inport  Port=4
  Corner and car centre 1 : Subsystem
  Corner and car centre 2 : Subsystem
  Demux : Demux
  Demux1 : Demux
  OR : Logic  Operator=OR  Inputs=8  IconShape=distinctive  AllPortsSameDT=off  OutDataTypeStr=boolean
  Subsystem10 : Subsystem
  Subsystem11 : Subsystem
  Subsystem3 : Subsystem
  Subsystem5 : Subsystem
  Subsystem6 : Subsystem
  Subsystem7 : Subsystem
  Subsystem8 : Subsystem
  Subsystem9 : Subsystem
  collided : Outport
  wires:
  pos1/1 -> Corner and car centre 1/2(pos1)
  Subsystem8/1(collided) -> OR/5
  Subsystem10/1(collided) -> OR/7
  Subsystem3/1(collided) -> OR/1
  Demux1/4 -> Subsystem11/3(v2cor4)
  Subsystem5/1(collided) -> OR/2
  Demux/1 -> Subsystem3/3(v1cor1)
  Subsystem11/1(collided) -> OR/8
  Subsystem7/1(collided) -> OR/4
  Corner and car centre 2/2(corners_v2) -> Demux1/1
  Demux1/3 -> Subsystem10/3(v2cor3)
  Demux/2 -> Subsystem5/3(v1cor2)
  psi1/1 -> Subsystem11/1(psi1), Subsystem10/1(psi1), Subsystem9/1(psi1), Subsystem8/1(psi1), Corner and car centre 1/1(psi1)
  Demux1/1 -> Subsystem8/3(v2cor1)
  Subsystem9/1(collided) -> OR/6
  OR/1 -> collided/1
  Demux1/2 -> Subsystem9/3(v2cor2)
  psi2/1 -> Subsystem7/1(psi2), Subsystem6/1(psi2), Subsystem5/1(psi2), Subsystem3/1(psi2), Corner and car centre 2/1(psi2)
  Corner and car centre 1/2(corners_v1) -> Demux/1
  Demux/3 -> Subsystem6/3(v1cor3)
  Corner and car centre 2/1(c2) -> Subsystem7/2(c2), Subsystem3/2(c2), Subsystem5/2(c2), Subsystem6/2(c2)
  pos2/1 -> Corner and car centre 2/2(pos2)
  Corner and car centre 1/1(c1) -> Subsystem11/2(c1), Subsystem10/2(c1), Subsystem9/2(c1), Subsystem8/2(c1)
  Subsystem6/1(collided) -> OR/3
  Demux/4 -> Subsystem7/3(v1cor4)

== system rlOvertakeTwoCars/Concatenate ==
  delta : Inport
  Matrix Concatenate : Concatenate
  AnF : Outport  VectorParamsAs1DForOutWhenUnconnected=off
  wires:
  Matrix Concatenate/1 -> AnF/1
  delta/1 -> Matrix Concatenate/2, Matrix Concatenate/1

== system rlOvertakeTwoCars/Concatenate Ego ==
  delta : Inport
  Matrix Concatenate : Concatenate
  AnF : Outport  VectorParamsAs1DForOutWhenUnconnected=off
  wires:
  Matrix Concatenate/1 -> AnF/1
  delta/1 -> Matrix Concatenate/2, Matrix Concatenate/1

== system rlOvertakeTwoCars/Final Trajectory Bird's-Eye Visualization Ego ==
  note: The subsystem displays the final vehicle trajectory in Bird's - Eye Scope
  Yaw : Inport
  YawRate : Inport  Port=2
  Info : Inport  Port=3
  Angular Velocity Conversion : aerolibconvert2/Angular Velocity Conversion  IU=rad/s  OU=deg/s
  Bus Selector1 : BusSelector  OutputSignals=InertFrm.Cg.Disp.X,InertFrm.Cg.Disp.Y,InertFrm.Cg.Vel.Xdot,InertFrm.Cg.Vel.Ydot
  Cuboid To 3D Simulation : drivingscenarioandsensors/Cuboid To 3D Simulation  SpecifyActorID=off  ActorIDToConvert=1  SimulateUsing=Interpreted execution
  Gain : Gain  Gain=-1
  Gain1 : Gain  Gain=-1
  Gain2 : Gain  Gain=-1
  MATLAB Function : MATLAB Function  TreatAsAtomicUnit=on
  Mux : Mux  Inputs=2
  Mux1 : Mux  Inputs=2
  Mux2 : Mux  Inputs=3
  Radians to Degrees : simulink_extras/Transformations/Radians to Degrees
  Rate Transition{,4..6} (4 alike) : RateTransition
  "Scenario Reader for Output " : drivingscenarioandsensors/Scenario Reader  Commented=through  ScenarioSource=From file  ScenarioFileName=testCorner_twoCars.mat  ScenarioVariableName=scenario  OutputCoordinateSystem=Vehicle coordinates  EgoVehicleSource=Input port  EgoVehicleActorID=1  OrientVehiclesOnRoad=off  OutputEgoVehiclePose=on  OutputEgoVehicleState=off  SampleTime=0.1  LaneBoundaryOutput=None  LaneBoundaryDistance=0:0.5:9.5  LaneBoundaryLocation=Center of lane markings  BusNameSource=Property  BusName=BusActors  BusNumActorsSource=Scenario  BusNumActors=100  BusName2Source=Auto  BusName2=BusLaneBoundaries  BusNumLaneBoundariesSource=Scenario  BusNumLaneBoundaries=10  BusName3Source=Auto  BusName3=BusEgoActor  BusName4Source=Auto  BusName4=BusEgoState  ShowCoordinateLabels=on  SimulateUsing=Interpreted execution
  Car1 : Outport
  wires:
  "Scenario Reader for Output "/1 -> Cuboid To 3D Simulation/1
  YawRate/1 -> Angular Velocity Conversion/1
  Yaw/1 -> Radians to Degrees/1
  Gain2/1 -> Rate Transition6/1
  Gain1/1 -> Rate Transition5/1
  Angular Velocity Conversion/1 -> Gain2/1
  Radians to Degrees/1 -> Gain1/1
  Info/1 -> Bus Selector1/1
  Bus Selector1/3 -> Mux1/1  "<Xdot>"
  Mux/1 -> Rate Transition/1
  Gain/1 -> Mux/2
  Bus Selector1/4 -> Mux1/2  "<Ydot>"
  Rate Transition5/1 -> MATLAB Function/3(yaw)
  Mux1/1 -> Rate Transition4/1
  Rate Transition4/1 -> MATLAB Function/2(vel)
  Bus Selector1/2 -> Gain/1  "<Y>"
  Bus Selector1/1 -> Mux/1  "<X>"
  Rate Transition/1 -> MATLAB Function/1(pos)
  Rate Transition6/1 -> MATLAB Function/4(yawRate)
  MATLAB Function/1(egoActor) -> "Scenario Reader for Output "/1
  Cuboid To 3D Simulation/1 -> Mux2/1
  Cuboid To 3D Simulation/2 -> Mux2/2
  Cuboid To 3D Simulation/3 -> Mux2/3
  Mux2/1 -> Car1/1

== system rlOvertakeTwoCars/Final Trajectory Bird's-Eye Visualization Lead ==
  note: The subsystem displays the final vehicle trajectory in Bird's - Eye Scope
  Yaw : Inport
  YawRate : Inport  Port=2
  Info : Inport  Port=3
  Angular Velocity Conversion : aerolibconvert2/Angular Velocity Conversion  IU=rad/s  OU=deg/s
  Bus Selector1 : BusSelector  OutputSignals=InertFrm.Cg.Disp.X,InertFrm.Cg.Disp.Y,InertFrm.Cg.Vel.Xdot,InertFrm.Cg.Vel.Ydot
  Cuboid To 3D Simulation : drivingscenarioandsensors/Cuboid To 3D Simulation  SpecifyActorID=off  ActorIDToConvert=1  SimulateUsing=Interpreted execution
  Gain : Gain  Gain=-1
  Gain1 : Gain  Gain=-1
  Gain2 : Gain  Gain=-1
  MATLAB Function : MATLAB Function  TreatAsAtomicUnit=on
  Mux : Mux  Inputs=2
  Mux1 : Mux  Inputs=2
  Mux2 : Mux  Inputs=3
  Radians to Degrees : simulink_extras/Transformations/Radians to Degrees
  Rate Transition{,4..6} (4 alike) : RateTransition
  "Scenario Reader for Output " : drivingscenarioandsensors/Scenario Reader  Commented=through  ScenarioSource=From file  ScenarioFileName=testCorner_twoCars.mat  ScenarioVariableName=scenario  OutputCoordinateSystem=Vehicle coordinates  EgoVehicleSource=Input port  EgoVehicleActorID=1  OrientVehiclesOnRoad=off  OutputEgoVehiclePose=on  OutputEgoVehicleState=off  SampleTime=0.1  LaneBoundaryOutput=None  LaneBoundaryDistance=0:0.5:9.5  LaneBoundaryLocation=Center of lane markings  BusNameSource=Property  BusName=BusActors  BusNumActorsSource=Scenario  BusNumActors=100  BusName2Source=Auto  BusName2=BusLaneBoundaries  BusNumLaneBoundariesSource=Scenario  BusNumLaneBoundaries=10  BusName3Source=Auto  BusName3=BusEgoActor  BusName4Source=Auto  BusName4=BusEgoState  ShowCoordinateLabels=on  SimulateUsing=Interpreted execution
  Car : Outport
  wires:
  "Scenario Reader for Output "/1 -> Cuboid To 3D Simulation/1
  YawRate/1 -> Angular Velocity Conversion/1
  Yaw/1 -> Radians to Degrees/1
  Gain2/1 -> Rate Transition6/1
  Gain1/1 -> Rate Transition5/1
  Angular Velocity Conversion/1 -> Gain2/1
  Radians to Degrees/1 -> Gain1/1
  Info/1 -> Bus Selector1/1
  Bus Selector1/3 -> Mux1/1  "<Xdot>"
  Mux/1 -> Rate Transition/1
  Gain/1 -> Mux/2
  Bus Selector1/4 -> Mux1/2  "<Ydot>"
  Rate Transition5/1 -> MATLAB Function/3(yaw)
  Mux1/1 -> Rate Transition4/1
  Rate Transition4/1 -> MATLAB Function/2(vel)
  Bus Selector1/2 -> Gain/1  "<Y>"
  Bus Selector1/1 -> Mux/1  "<X>"
  Rate Transition/1 -> MATLAB Function/1(pos)
  Rate Transition6/1 -> MATLAB Function/4(yawRate)
  MATLAB Function/1(egoActor) -> "Scenario Reader for Output "/1
  Mux2/1 -> Car/1
  Cuboid To 3D Simulation/1 -> Mux2/1
  Cuboid To 3D Simulation/2 -> Mux2/2
  Cuboid To 3D Simulation/3 -> Mux2/3

== system rlOvertakeTwoCars/MPC Based Controller ==
  note: The 'Dead Zone' blocks is used to ensure that the pedal command is zero.
  note: This 2-D Lookup Table was created using a for-loop and then normalizing. This is required because the output of the MPC controller is acceleration (m/s^2), but the powertrain model uses pedal commands from 0-1.
      |
      | Here are the steps in the script to create the table:
      |
      | 1.) The for-loop is used to calculate the required torque (Nm) from the powertrain.
      | 2.) The positive torque values are normalized based on peak positive motor torque, and the negative torques are normalized based on the peak brake pressure. This results in a pedal map with values of -1 to 1.
      |
      | This map required two values to be calibrated.
      |
      | This is a simple linearized map, but this can be altered for better drivability.
  Pose : Inport
  VelRef : Inport  Port=2
  VelFdbk : Inport  Port=3
  1-D Lookup Table1 : Lookup_n-D  NumberOfTableDimensions=1  BreakpointsForDimension1=gradbp1  Table=curvature1  InterpMethod=Cubic spline  ExtrapMethod=Clip  InternalRulePriority=Speed  RndMeth=Simplest
  Integrator : Integrator
  Path Following Control System MPC : mpcadaslib/Path Following Control System  VariantControl=Variant2  ModelType=Use vehicle parameters  VehicleMass=2000  VehicleYawInertia=4000  LengthToFront=1.4  LengthToRear=1.6  FrontTireStiffness=12e3  RearTireStiffness=11e3  AccelTimeConstant=0.5  EgoModelMatrixA=[-2,zeros(1,3);1,zeros(1,3);zeros(1,2),-4.4021,-12.4603;zeros(1,2),1.3913,-5.1868]  EgoModelMatrixB=[2,zeros(1,3);zeros(1,2),24.1270,15.8609]'  EgoModelMatrixC=[zeros(3,1),eye(3)]  InitialLongVel=v_o1  TransportLag=0  spaceCtrl=off  DefaultSpacing=10  MinSteering=umin  umin_ext=off  MaxSteering=umax  umax_ext=off  MinAcceleration=amin  amin_ext=off  MaxAcceleration=amax  amax_ext=off  Ts=Ts  PredictionHorizon=pred_horizon  ControlHorizon=cont_horizon  LongWeight=w_veltrack  LateralWeight=w_laterror  AccelRateWeight=w_dax  SteerRateWeight=w_dphi  suboptimal=off  maxiter=10  datatypeopt=double  optmode=off  trackmode=off
      link override Longitudinal velocity must be positive: enabled=on
  Pedal map : Subsystem
  Sensor Dynamics : Subsystem
  Terminator : Terminator
  WheelSteeringAngle : Outport
  AccelCmd : Outport  Port=2
  DecelCmd : Outport  Port=3
  wires:
  Path Following Control System MPC/1 -> Pedal map/2(a)  "a"
  Pedal map/2(Out2) -> DecelCmd/1
  Sensor Dynamics/2(Relative yaw angle) -> Path Following Control System MPC/5
  VelRef/1 -> Path Following Control System MPC/1
  [yawrate1] -> Sensor Dynamics/4(Yaw rate)
  [ydot1] -> Sensor Dynamics/3(Lateral velocity)
  Path Following Control System MPC/2 -> WheelSteeringAngle/1
  1-D Lookup Table1/1 -> Sensor Dynamics/1(Current curvature), Path Following Control System MPC/3  "rho"
  Pedal map/1(Out1) -> AccelCmd/1
  Sensor Dynamics/1(Lateral deviation) -> Path Following Control System MPC/4
  Integrator/1 -> 1-D Lookup Table1/1  "distance"
  VelFdbk/1 -> Pedal map/1(vx), Path Following Control System MPC/2, Integrator/1, Sensor Dynamics/2(Longitudinal velocity)  "vx"
  Pose/1 -> Terminator/1
